simulink model "vision_loop_meme_interface_hrn"  (R2014b)
settings: Solver=FixedStepDiscrete  StartTime=t0  StopTime=tFinal  FixedStep=dt  RelTol=1e-3
values from neighbouring files (symbols this model uses):
  cam_cam1_pos_in_lander = [0 0 -0.5]'    [csc_cam_camera_system_init.m]
undefined symbols (not defined in the file or in its folder): cam_cam1_lander_dcm, cam_cam1_lander_quat, cam_process_pair_counter, cam_take_image_counter, cam_use_meme_flag, csc_cam_camera_system, csc_cam_camera_system_lib, csc_cmg_camera_geometry, csc_cmg_camera_geometry_lib, ini_tgt_landing_mcmf_pos, KF_DT
undefined symbols (not defined in the file): cam_kir_image_size, cam_kir_intrinsics
libraries: util_quat_lib x24, util_frame_rotation_lib x8, util_info_lib x3, csu_cis_camera_image_sim_lib x3, simulink x1, csu_kir_image_request_lib x1, csc_fdm_feature_detection_matching_lib x1, csu_kfd_orb_feature_matching_lib x1, csu_und_unduplicate_lib x1
settings Model: Creator=escrane  LastModifiedBy=mstewart
settings DebuggingCC: UnderspecifiedInitializationDetection=Classic  MergeDetectMultiDrivingBlocksExec=none  StateNameClashWarn=warning

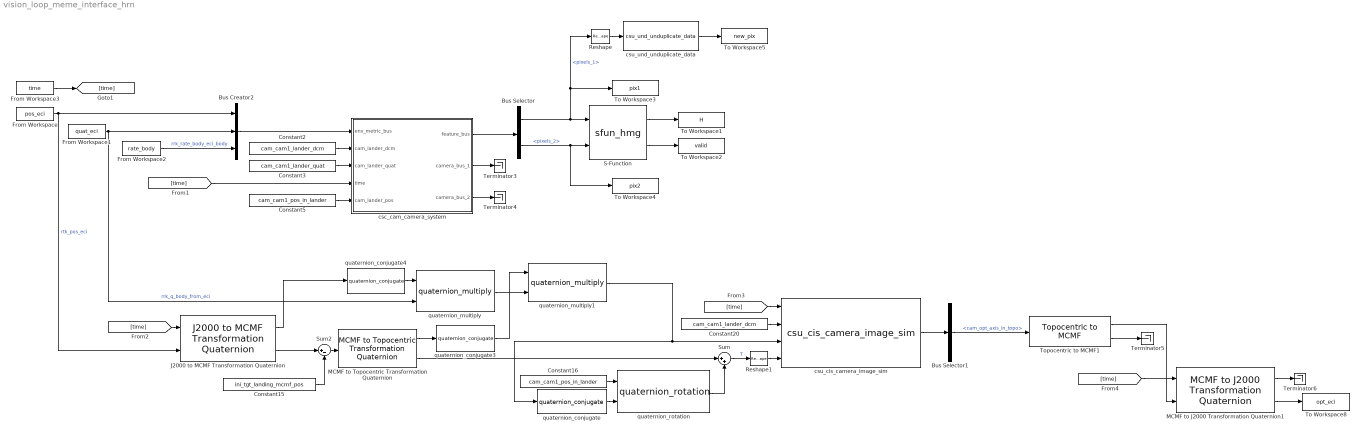
== system vision_loop_meme_interface_hrn ==
  Bus Creator2 : BusCreator  Inputs=3
  Bus Selector : BusSelector  OutputSignals=pixels_1,pixels_2
  Bus Selector1 : BusSelector  OutputSignals=cam_opt_axis_in_topo
  Constant15 : Constant  Value=ini_tgt_landing_mcmf_pos
  Constant16 : Constant  Value=cam_cam1_pos_in_lander
  Constant2 : Constant  Value=cam_cam1_lander_dcm
  Constant20 : Constant  Value=cam_cam1_lander_dcm
  Constant3 : Constant  Value=cam_cam1_lander_quat
  Constant5 : Constant  Value=cam_cam1_pos_in_lander
  From Workspace : FromWorkspace  VariableName=pos_eci  SampleTime=0
  From Workspace1 : FromWorkspace  VariableName=quat_eci  SampleTime=0
  From Workspace2 : FromWorkspace  VariableName=rate_body  SampleTime=0
  From Workspace3 : FromWorkspace  VariableName=time  SampleTime=0
  J2000 to MCMF Transformation Quaternion : util_frame_rotation_lib/J2000 to MCMF  Transformation Quaternion  SystemSampleTime=-1
  MCMF to J2000 Transformation Quaternion1 : util_frame_rotation_lib/MCMF to J2000  Transformation Quaternion
  MCMF to Topocentric Transformation Quaternion : util_frame_rotation_lib/MCMF to Topocentric  Transformation Quaternion  SystemSampleTime=-1
  Reshape : Reshape
  Reshape1 : Reshape  OutputDimensionality=Column vector (2-D)
  S-Function : S-Function  FunctionName=sfun_hmg  Parameters=2  EnableBusSupport=off
  Sum : Sum  Inputs=|++
  Sum2 : Sum  Inputs=|+-
  Terminator{3..6} (4 alike) : Terminator
  To Workspace1 : ToWorkspace  VariableName=H  SaveFormat=Timeseries  SampleTime=-1
  To Workspace2 : ToWorkspace  VariableName=valid  SaveFormat=Timeseries  SampleTime=-1
  To Workspace3 : ToWorkspace  VariableName=pix1  SaveFormat=Timeseries  SampleTime=-1
  To Workspace4 : ToWorkspace  VariableName=pix2  SaveFormat=Timeseries  SampleTime=-1
  To Workspace5 : ToWorkspace  VariableName=new_pix  SaveFormat=Timeseries  SampleTime=-1
  To Workspace8 : ToWorkspace  VariableName=opt_eci  SaveFormat=Timeseries  SampleTime=-1
  Topocentric to MCMF1 : util_frame_rotation_lib/Topocentric to MCMF  SystemSampleTime=-1
  csc_cam_camera_system : Subsystem  AncestorBlock=csc_cam_camera_system_lib/csc_cam_camera_system  SystemSampleTime=KF_DT
  csu_cis_camera_image_sim : csu_cis_camera_image_sim_lib/csu_cis_camera_image_sim
  csu_und_unduplicate_data : csu_und_unduplicate_lib/csu_und_unduplicate_data  initial_compare=0
  quaternion_conjugate : util_quat_lib/quaternion_conjugate  SystemSampleTime=-1
  quaternion_conjugate3 : util_quat_lib/quaternion_conjugate  SystemSampleTime=-1
  quaternion_conjugate4 : util_quat_lib/quaternion_conjugate  SystemSampleTime=-1
  quaternion_multiply : util_quat_lib/quaternion_multiply  SystemSampleTime=-1
  quaternion_multiply1 : util_quat_lib/quaternion_multiply  SystemSampleTime=-1
  quaternion_rotation : util_quat_lib/quaternion_rotation  SystemSampleTime=-1
  wires:
  Constant2/1 -> csc_cam_camera_system/2(cam_lander_dcm)
  Constant3/1 -> csc_cam_camera_system/3(cam_lander_quat)
  Constant5/1 -> csc_cam_camera_system/5(cam_lander_pos)
  [time] -> csc_cam_camera_system/4(time)
  From Workspace/1 -> J2000 to MCMF Transformation Quaternion/2, Bus Creator2/1  "rtk_pos_eci"
  Bus Creator2/1 -> csc_cam_camera_system/1(env_metric_bus)
  From Workspace1/1 -> Bus Creator2/2, quaternion_multiply/2  "rrk_q_body_from_eci"
  csc_cam_camera_system/2(camera_bus_1) -> Terminator3/1
  csc_cam_camera_system/3(camera_bus_2) -> Terminator4/1
  Sum2/1 -> MCMF to Topocentric Transformation Quaternion/1
  J2000 to MCMF Transformation Quaternion/2 -> Sum2/1
  Constant15/1 -> Sum2/2
  [time] -> J2000 to MCMF Transformation Quaternion/1
  J2000 to MCMF Transformation Quaternion/1 -> quaternion_conjugate4/1
  quaternion_conjugate4/1 -> quaternion_multiply/1
  quaternion_multiply/1 -> quaternion_multiply1/2
  quaternion_conjugate3/1 -> quaternion_multiply1/1
  MCMF to Topocentric Transformation Quaternion/1 -> quaternion_conjugate3/1
  quaternion_conjugate/1 -> quaternion_rotation/2
  MCMF to Topocentric Transformation Quaternion/2 -> Sum/1
  quaternion_multiply1/1 -> csu_cis_camera_image_sim/3, quaternion_conjugate/1
  Constant16/1 -> quaternion_rotation/1
  quaternion_rotation/1 -> Sum/2
  Sum/1 -> Reshape1/1  "T"
  Reshape1/1 -> csu_cis_camera_image_sim/4
  Constant20/1 -> csu_cis_camera_image_sim/2
  [time] -> csu_cis_camera_image_sim/1
  csu_cis_camera_image_sim/1 -> Bus Selector1/1
  Topocentric to MCMF1/1 -> MCMF to J2000 Transformation Quaternion1/2
  [time] -> MCMF to J2000 Transformation Quaternion1/1
  MCMF to J2000 Transformation Quaternion1/2 -> To Workspace8/1
  Topocentric to MCMF1/2 -> Terminator5/1
  MCMF to J2000 Transformation Quaternion1/1 -> Terminator6/1
  Bus Selector1/1 -> Topocentric to MCMF1/1  "<cam_opt_axis_in_topo>"
  Bus Selector/1 -> To Workspace3/1, Reshape/1, S-Function/1  "<pixels_1>"
  Bus Selector/2 -> To Workspace4/1, S-Function/2  "<pixels_2>"
  csc_cam_camera_system/1(feature_bus) -> Bus Selector/1
  S-Function/1 -> To Workspace1/1
  S-Function/2 -> To Workspace2/1
  From Workspace2/1 -> Bus Creator2/3  "rrk_rate_body_eci_body"
  From Workspace3/1 -> [time]
  Reshape/1 -> csu_und_unduplicate_data/1
  csu_und_unduplicate_data/1 -> To Workspace5/1

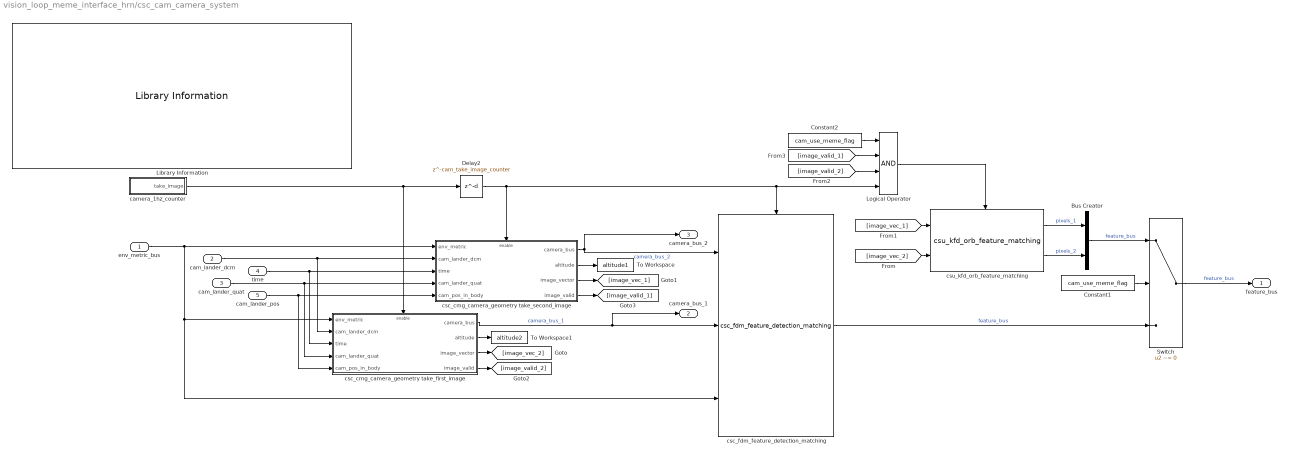
== system vision_loop_meme_interface_hrn/csc_cam_camera_system ==
  env_metric_bus : Inport
  cam_lander_dcm : Inport  Port=2
  cam_lander_quat : Inport  Port=3
  time : Inport  Port=4
  cam_lander_pos : Inport  Port=5
  Bus Creator : BusCreator  Inputs=2
  Constant1 : Constant  Value=cam_use_meme_flag
  Constant2 : Constant  Value=cam_use_meme_flag
  Delay2 : Delay  DelayLength=cam_take_image_counter
  Library Information : util_info_lib/Library Information  owner='NONE'
  Logical Operator : Logic  Inputs=4  AllPortsSameDT=off  OutDataTypeStr=boolean
  Switch : Switch  Criteria=u2 ~= 0
  To Workspace : ToWorkspace  VariableName=altitude1  SaveFormat=Timeseries  SampleTime=-1
  To Workspace1 : ToWorkspace  VariableName=altitude2  SaveFormat=Timeseries  SampleTime=-1
  camera_1hz_counter : Subsystem  TreatAsAtomicUnit=on
  csc_cmg_camera_geometry take_first_image : Subsystem  AncestorBlock=csc_cmg_camera_geometry_lib/csc_cmg_camera_geometry
  csc_cmg_camera_geometry take_second_image : Subsystem  AncestorBlock=csc_cmg_camera_geometry_lib/csc_cmg_camera_geometry
  csc_fdm_feature_detection_matching : csc_fdm_feature_detection_matching_lib/csc_fdm_feature_detection_matching
  csu_kfd_orb_feature_matching : csu_kfd_orb_feature_matching_lib/csu_kfd_orb_feature_matching  size=cam_kir_image_size
  feature_bus : Outport
  camera_bus_1 : Outport  Port=2
  camera_bus_2 : Outport  Port=3
  wires:
  Constant2/1 -> Logical Operator/1
  [image_valid_2] -> Logical Operator/3
  [image_valid_1] -> Logical Operator/2
  csc_cmg_camera_geometry take_first_image/1(camera_bus) -> camera_bus_1/1, csc_fdm_feature_detection_matching/2  "camera_bus_1"
  Delay2/1 -> csc_cmg_camera_geometry take_second_image/Enable, Logical Operator/4, csc_fdm_feature_detection_matching/Enable
  env_metric_bus/1 -> csc_fdm_feature_detection_matching/3, csc_cmg_camera_geometry take_first_image/1(env_metric), csc_cmg_camera_geometry take_second_image/1(env_metric)
  camera_1hz_counter/1(take_image) -> Delay2/1, csc_cmg_camera_geometry take_first_image/Enable
  csc_cmg_camera_geometry take_second_image/1(camera_bus) -> camera_bus_2/1, csc_fdm_feature_detection_matching/1  "camera_bus_2"
  cam_lander_dcm/1 -> csc_cmg_camera_geometry take_second_image/2(cam_lander_dcm), csc_cmg_camera_geometry take_first_image/2(cam_lander_dcm)
  cam_lander_quat/1 -> csc_cmg_camera_geometry take_first_image/4(cam_lander_quat), csc_cmg_camera_geometry take_second_image/4(cam_lander_quat)
  time/1 -> csc_cmg_camera_geometry take_second_image/3(time), csc_cmg_camera_geometry take_first_image/3(time)
  csc_cmg_camera_geometry take_second_image/3(image_vector) -> [image_vec_1]
  csc_cmg_camera_geometry take_second_image/4(image_valid) -> [image_valid_1]
  csc_cmg_camera_geometry take_first_image/4(image_valid) -> [image_valid_2]
  [image_vec_1] -> csu_kfd_orb_feature_matching/1
  [image_vec_2] -> csu_kfd_orb_feature_matching/2
  Logical Operator/1 -> csu_kfd_orb_feature_matching/Enable
  csu_kfd_orb_feature_matching/2 -> Bus Creator/2  "pixels_2"
  csu_kfd_orb_feature_matching/1 -> Bus Creator/1  "pixels_1"
  Bus Creator/1 -> Switch/1  "feature_bus"
  Switch/1 -> feature_bus/1  "feature_bus"
  csc_fdm_feature_detection_matching/1 -> Switch/3  "feature_bus"
  Constant1/1 -> Switch/2
  cam_lander_pos/1 -> csc_cmg_camera_geometry take_first_image/5(cam_pos_in_body), csc_cmg_camera_geometry take_second_image/5(cam_pos_in_body)
  csc_cmg_camera_geometry take_second_image/2(altitude) -> To Workspace/1
  csc_cmg_camera_geometry take_first_image/3(image_vector) -> [image_vec_2]
  csc_cmg_camera_geometry take_first_image/2(altitude) -> To Workspace1/1

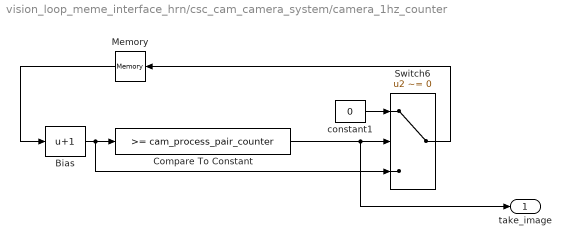
== system vision_loop_meme_interface_hrn/csc_cam_camera_system/camera_1hz_counter ==
  Bias : Bias  Bias=1
  Compare To Constant : simulink/Logic and Bit Operations/Compare To Constant  relop=>=  const=cam_process_pair_counter  OutDataTypeStr=uint8
  Memory : Memory  X0=cam_process_pair_counter  InheritSampleTime=on
  Switch6 : Switch  Criteria=u2 ~= 0  InputSameDT=on
  constant1 : Constant  Value=0
  take_image : Outport
  wires:
  constant1/1 -> Switch6/1
  Bias/1 -> Compare To Constant/1, Switch6/3
  Compare To Constant/1 -> Switch6/2, take_image/1
  Switch6/1 -> Memory/1
  Memory/1 -> Bias/1

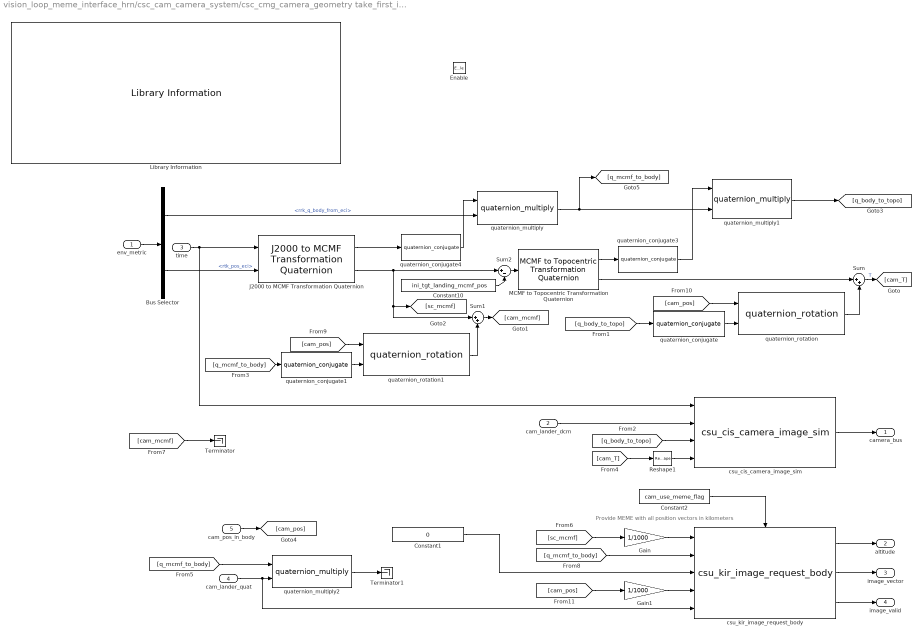
== system vision_loop_meme_interface_hrn/csc_cam_camera_system/csc_cmg_camera_geometry take_first_image ==
  note: Provide MEME with all position vectors in kilometers
  env_metric : Inport
  cam_lander_dcm : Inport  Port=2
  time : Inport  Port=3
  cam_lander_quat : Inport  Port=4
  cam_pos_in_body : Inport  Port=5
  Enable : EnablePort
  Bus Selector : BusSelector  OutputSignals=rrk_q_body_from_eci,rtk_pos_eci
  Constant1 : Constant  Value=0  OutDataTypeStr=int32
  Constant10 : Constant  Value=ini_tgt_landing_mcmf_pos
  Constant2 : Constant  Value=cam_use_meme_flag
  Gain : Gain  Gain=1/1000
  Gain1 : Gain  Gain=1/1000
  J2000 to MCMF Transformation Quaternion : util_frame_rotation_lib/J2000 to MCMF  Transformation Quaternion  SystemSampleTime=-1
  Library Information : util_info_lib/Library Information  owner='NONE'
  MCMF to Topocentric Transformation Quaternion : util_frame_rotation_lib/MCMF to Topocentric  Transformation Quaternion  SystemSampleTime=-1
  Reshape1 : Reshape  OutputDimensionality=Column vector (2-D)
  Sum : Sum  Inputs=|++
  Sum1 : Sum  Inputs=|++
  Sum2 : Sum  Inputs=|+-
  Terminator : Terminator
  Terminator1 : Terminator
  csu_cis_camera_image_sim : csu_cis_camera_image_sim_lib/csu_cis_camera_image_sim
  csu_kir_image_request_body : csu_kir_image_request_lib/csu_kir_image_request_body  size=cam_kir_image_size  intrinsics=cam_kir_intrinsics
      link override S-Function: Parameters=192 168 1 12 5000
  quaternion_conjugate{,1,3..4} (4 alike) : util_quat_lib/quaternion_conjugate  SystemSampleTime=-1
  quaternion_multiply : util_quat_lib/quaternion_multiply  SystemSampleTime=-1
  quaternion_multiply1 : util_quat_lib/quaternion_multiply  SystemSampleTime=-1
  quaternion_multiply2 : util_quat_lib/quaternion_multiply  SystemSampleTime=-1
  quaternion_rotation : util_quat_lib/quaternion_rotation  SystemSampleTime=-1
  quaternion_rotation1 : util_quat_lib/quaternion_rotation  SystemSampleTime=-1
  camera_bus : Outport
  altitude : Outport  Port=2
  image_vector : Outport  Port=3
  image_valid : Outport  Port=4
  wires:
  Gain1/1 -> csu_kir_image_request_body/4
  [cam_pos] -> Gain1/1
  cam_pos_in_body/1 -> [cam_pos]
  [cam_mcmf] -> Terminator/1
  Constant2/1 -> csu_kir_image_request_body/Enable
  Reshape1/1 -> csu_cis_camera_image_sim/4
  csu_cis_camera_image_sim/1 -> camera_bus/1
  [q_body_to_topo] -> csu_cis_camera_image_sim/3
  cam_lander_dcm/1 -> csu_cis_camera_image_sim/2
  Sum2/1 -> MCMF to Topocentric Transformation Quaternion/1
  J2000 to MCMF Transformation Quaternion/2 -> Sum1/1, [sc_mcmf], Sum2/1
  Constant10/1 -> Sum2/2
  csu_kir_image_request_body/2 -> image_vector/1
  Constant1/1 -> csu_kir_image_request_body/3
  [sc_mcmf] -> Gain/1
  [q_mcmf_to_body] -> quaternion_multiply2/1
  Sum1/1 -> [cam_mcmf]
  quaternion_rotation1/1 -> Sum1/2
  [q_mcmf_to_body] -> quaternion_conjugate1/1
  quaternion_conjugate1/1 -> quaternion_rotation1/2
  [cam_pos] -> quaternion_rotation1/1
  time/1 -> J2000 to MCMF Transformation Quaternion/1, csu_cis_camera_image_sim/1
  [cam_T] -> Reshape1/1
  J2000 to MCMF Transformation Quaternion/1 -> quaternion_conjugate4/1
  quaternion_conjugate4/1 -> quaternion_multiply/1
  Bus Selector/1 -> quaternion_multiply/2  "<rrk_q_body_from_eci>"
  quaternion_multiply/1 -> quaternion_multiply1/2, [q_mcmf_to_body]
  quaternion_conjugate3/1 -> quaternion_multiply1/1
  MCMF to Topocentric Transformation Quaternion/1 -> quaternion_conjugate3/1
  quaternion_conjugate/1 -> quaternion_rotation/2
  quaternion_multiply1/1 -> [q_body_to_topo]
  MCMF to Topocentric Transformation Quaternion/2 -> Sum/1
  env_metric/1 -> Bus Selector/1
  Bus Selector/2 -> J2000 to MCMF Transformation Quaternion/2  "<rtk_pos_eci>"
  [q_body_to_topo] -> quaternion_conjugate/1
  [cam_pos] -> quaternion_rotation/1
  quaternion_rotation/1 -> Sum/2
  Sum/1 -> [cam_T]  "T"
  Gain/1 -> csu_kir_image_request_body/1
  cam_lander_quat/1 -> csu_kir_image_request_body/5, quaternion_multiply2/2
  [q_mcmf_to_body] -> csu_kir_image_request_body/2
  quaternion_multiply2/1 -> Terminator1/1
  csu_kir_image_request_body/3 -> image_valid/1
  csu_kir_image_request_body/1 -> altitude/1

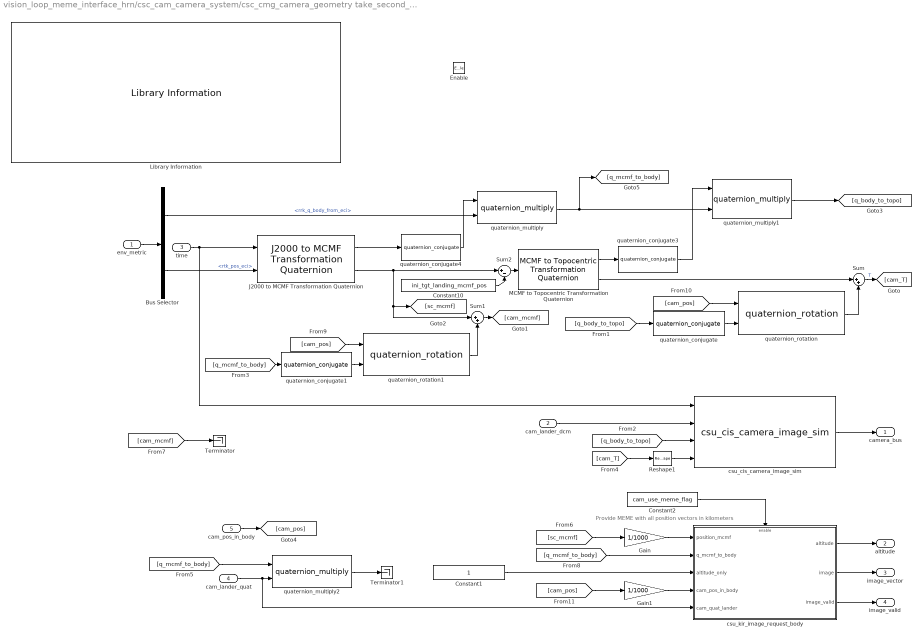
== system vision_loop_meme_interface_hrn/csc_cam_camera_system/csc_cmg_camera_geometry take_second_image ==
  note: Provide MEME with all position vectors in kilometers
  env_metric : Inport
  cam_lander_dcm : Inport  Port=2
  time : Inport  Port=3
  cam_lander_quat : Inport  Port=4
  cam_pos_in_body : Inport  Port=5
  Enable : EnablePort
  Bus Selector : BusSelector  OutputSignals=rrk_q_body_from_eci,rtk_pos_eci
  Constant1 : Constant  OutDataTypeStr=int32
  Constant10 : Constant  Value=ini_tgt_landing_mcmf_pos
  Constant2 : Constant  Value=cam_use_meme_flag
  Gain : Gain  Gain=1/1000
  Gain1 : Gain  Gain=1/1000
  J2000 to MCMF Transformation Quaternion : util_frame_rotation_lib/J2000 to MCMF  Transformation Quaternion  SystemSampleTime=-1
  Library Information : util_info_lib/Library Information  owner='NONE'
  MCMF to Topocentric Transformation Quaternion : util_frame_rotation_lib/MCMF to Topocentric  Transformation Quaternion  SystemSampleTime=-1
  Reshape1 : Reshape  OutputDimensionality=Column vector (2-D)
  Sum : Sum  Inputs=|++
  Sum1 : Sum  Inputs=|++
  Sum2 : Sum  Inputs=|+-
  Terminator : Terminator
  Terminator1 : Terminator
  csu_cis_camera_image_sim : csu_cis_camera_image_sim_lib/csu_cis_camera_image_sim
  csu_kir_image_request_body : Subsystem  AncestorBlock=csu_kir_image_request_lib/csu_kir_image_request_body  mask{size=cam_kir_image_size, intrinsics=cam_kir_intrinsics}
      mask prompts: size "Image Size [cols rows]"; intrinsics "Camera Intrinsics [f pixel_size]"
  quaternion_conjugate{,1,3..4} (4 alike) : util_quat_lib/quaternion_conjugate  SystemSampleTime=-1
  quaternion_multiply : util_quat_lib/quaternion_multiply  SystemSampleTime=-1
  quaternion_multiply1 : util_quat_lib/quaternion_multiply  SystemSampleTime=-1
  quaternion_multiply2 : util_quat_lib/quaternion_multiply  SystemSampleTime=-1
  quaternion_rotation : util_quat_lib/quaternion_rotation  SystemSampleTime=-1
  quaternion_rotation1 : util_quat_lib/quaternion_rotation  SystemSampleTime=-1
  camera_bus : Outport
  altitude : Outport  Port=2
  image_vector : Outport  Port=3
  image_valid : Outport  Port=4
  wires:
  Gain1/1 -> csu_kir_image_request_body/4(cam_pos_in_body)
  [cam_pos] -> Gain1/1
  cam_pos_in_body/1 -> [cam_pos]
  [cam_mcmf] -> Terminator/1
  Constant2/1 -> csu_kir_image_request_body/Enable
  Reshape1/1 -> csu_cis_camera_image_sim/4
  csu_cis_camera_image_sim/1 -> camera_bus/1
  [q_body_to_topo] -> csu_cis_camera_image_sim/3
  cam_lander_dcm/1 -> csu_cis_camera_image_sim/2
  Sum2/1 -> MCMF to Topocentric Transformation Quaternion/1
  J2000 to MCMF Transformation Quaternion/2 -> Sum1/1, [sc_mcmf], Sum2/1
  Constant10/1 -> Sum2/2
  csu_kir_image_request_body/2(image) -> image_vector/1
  [sc_mcmf] -> Gain/1
  [q_mcmf_to_body] -> quaternion_multiply2/1
  Sum1/1 -> [cam_mcmf]
  quaternion_rotation1/1 -> Sum1/2
  [q_mcmf_to_body] -> quaternion_conjugate1/1
  quaternion_conjugate1/1 -> quaternion_rotation1/2
  [cam_pos] -> quaternion_rotation1/1
  time/1 -> J2000 to MCMF Transformation Quaternion/1, csu_cis_camera_image_sim/1
  [cam_T] -> Reshape1/1
  J2000 to MCMF Transformation Quaternion/1 -> quaternion_conjugate4/1
  quaternion_conjugate4/1 -> quaternion_multiply/1
  Bus Selector/1 -> quaternion_multiply/2  "<rrk_q_body_from_eci>"
  quaternion_multiply/1 -> quaternion_multiply1/2, [q_mcmf_to_body]
  quaternion_conjugate3/1 -> quaternion_multiply1/1
  MCMF to Topocentric Transformation Quaternion/1 -> quaternion_conjugate3/1
  quaternion_conjugate/1 -> quaternion_rotation/2
  quaternion_multiply1/1 -> [q_body_to_topo]
  MCMF to Topocentric Transformation Quaternion/2 -> Sum/1
  env_metric/1 -> Bus Selector/1
  Bus Selector/2 -> J2000 to MCMF Transformation Quaternion/2  "<rtk_pos_eci>"
  [q_body_to_topo] -> quaternion_conjugate/1
  [cam_pos] -> quaternion_rotation/1
  quaternion_rotation/1 -> Sum/2
  Sum/1 -> [cam_T]  "T"
  Gain/1 -> csu_kir_image_request_body/1(position_mcmf)
  cam_lander_quat/1 -> csu_kir_image_request_body/5(cam_quat_lander), quaternion_multiply2/2
  [q_mcmf_to_body] -> csu_kir_image_request_body/2(q_mcmf_to_body)
  quaternion_multiply2/1 -> Terminator1/1
  csu_kir_image_request_body/3(image_valid) -> image_valid/1
  csu_kir_image_request_body/1(altitude) -> altitude/1
  Constant1/1 -> csu_kir_image_request_body/3(altitude_only)

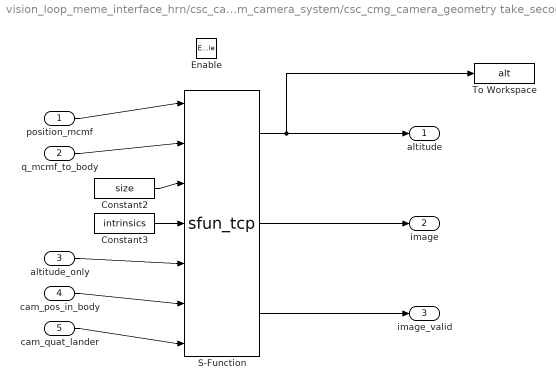
== system vision_loop_meme_interface_hrn/csc_cam_camera_system/csc_cmg_camera_geometry take_second_image/csu_kir_image_request_body ==
  position_mcmf : Inport
  q_mcmf_to_body : Inport  Port=2
  altitude_only : Inport  Port=3
  cam_pos_in_body : Inport  Port=4
  cam_quat_lander : Inport  Port=5
  Enable : EnablePort
  Constant2 : Constant  Value=size
  Constant3 : Constant  Value=intrinsics
  S-Function : S-Function  FunctionName=sfun_tcp  Parameters=192 168 1 12 5000  EnableBusSupport=off
  To Workspace : ToWorkspace  VariableName=alt  SaveFormat=Timeseries  SampleTime=-1
  altitude : Outport
  image : Outport  Port=2  InitialOutput=0
  image_valid : Outport  Port=3  InitialOutput=0
  wires:
  cam_quat_lander/1 -> S-Function/7
  cam_pos_in_body/1 -> S-Function/6
  S-Function/2 -> image/1
  Constant3/1 -> S-Function/4
  Constant2/1 -> S-Function/3
  altitude_only/1 -> S-Function/5
  q_mcmf_to_body/1 -> S-Function/2
  position_mcmf/1 -> S-Function/1
  S-Function/1 -> To Workspace/1, altitude/1
  S-Function/3 -> image_valid/1
